simulink model "QAM_model1"  (Simulink 7.6)
settings: Solver=FixedStepDiscrete  SolverMode=SingleTasking  StartTime=0.0  StopTime=1  FixedStep=Ts  RelTol=1e-3  AbsTol=1e-6
PreLoadFcn:
  | fs=100000; Ts=1/fs; R=1000; T=1/R; fc=10000; M=16; A=20*sqrt(T/2);
undefined symbols (not defined in the file): get
libraries: commsink2 x2, commfilt2 x2, simulink x2, commrandsrc2 x1
settings Model: Creator=Lab220  LastModifiedBy=Sílvio
settings DataIOCC: LimitDataPoints=off  SignalLoggingName=sigsOut
settings OptimizationCC: BooleanDataType=off
settings DebuggingCC: SaveWithParameterizedLinksMsg=none  SignalResolutionControl=TryResolveAllWithWarning  SolverPrmCheckMsg=none  MultiTaskDSMMsg=warning  MultiTaskCondExecSysMsg=none  StrictBusMsg=None
settings HardwareCC: TargetUnknown=on
settings RTWCC: TemplateMakefile=grt_unix.tmf  IncludeERTFirstTime=on
settings GRTTargetCC: ModelReferenceCompliant=off  MatFileLogging=off

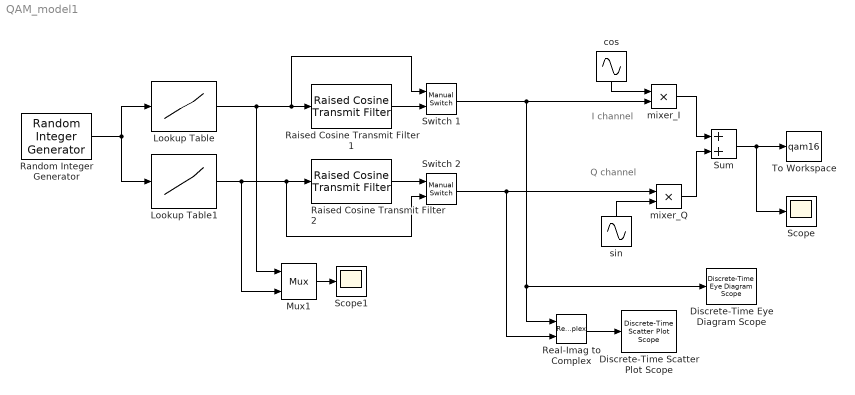
== system QAM_model1 ==
  note: I channel
  note: Q channel
  Discrete-Time Eye Diagram Scope : commsink2/Discrete-Time Eye Diagram Scope  Tag=EyeDiagram  SystemSampleTime=-1  sampPerSymb=100  offsetEye=0  symbPerTrace=2  numTraces=100  numNewFrames=4  LineStyles=-  LineColors=b  dupPoints=on  fading=on  render=on  AxisGrid=on  yMin=-4  yMax=4  inphaseLabel=In-phase Amplitude  quadratureLabel=Quadrature Amplitude  openScopeAtSimStart=on  dispDiagram=In-phase Only  FrameNumber=off  FigPos=get(0,'defaultfigureposition');  figTitle=Eye Diagram  block_type_=eye  numLinesMax=8
  Discrete-Time Scatter Plot Scope : commsink2/Discrete-Time Scatter Plot Scope  Tag=ScatterPlot  SystemSampleTime=-1  sampPerSymb=fs/R  offsetEye=0  numTraces=100  numNewFrames=100  LineMarkers=.  LineColors=b  fading=on  render=on  AxisGrid=on  xMin=-4  xMax=4  yMin=-4  yMax=4  inphaseLabel=In-phase Amplitude  quadratureLabel=Quadrature Amplitude  openScopeAtSimStart=on  FrameNumber=off  FigPos=get(0,'defaultfigureposition');  figTitle=Scatter Plot  numLinesMax=8  block_type_=scatter
  Lookup Table : Lookup_n-D  NumberOfTableDimensions=1  BreakpointsForDimension1=[0:15]  Table=[-3 -3 -3 -3 -1 -1 -1 -1 3 3 3 3 1 1 1 1]  InputSameDT=on
  Lookup Table1 : Lookup_n-D  NumberOfTableDimensions=1  BreakpointsForDimension1=[0:15]  Table=[-3 -1 3 1 -3 -1 3 1 -3 -1 3 1 -3 -1 3 1]  InputSameDT=on
  Mux1 : Mux  Inputs=2
  Raised Cosine Transmit Filter 1 : commfilt2/Raised Cosine Transmit Filter  DialogController=dspDDGCreate  DialogControllerArgs=DataTag1  SystemSampleTime=-1  filtType=Normal  D=4  R=0.5  sampMode=Mute  saveAsFlag=0  N=100  framing=Maintain input frame size  checkGain=Normalized  filterGain=1  checkCoeff=off  variableName=rcTxFilt  launchFVT=off  roundingMode=Floor  overflowMode=off
  Raised Cosine Transmit Filter 2 : commfilt2/Raised Cosine Transmit Filter  DialogController=dspDDGCreate  DialogControllerArgs=DataTag3  SystemSampleTime=-1  filtType=Normal  D=4  R=0.5  sampMode=Mute  saveAsFlag=0  N=100  framing=Maintain input frame size  checkGain=Normalized  filterGain=1  checkCoeff=off  variableName=rcTxFilt1  launchFVT=off  roundingMode=Floor  overflowMode=off
  Random Integer Generator : commrandsrc2/Random Integer Generator  SystemSampleTime=-1  mul=M  seed=randseed  Ts=T  frameBased=off  sampPerFrame=1  orient=off  outDataType=double
  Real-Imag to Complex : RealImagToComplex
  Scope : Scope
      settings: TickLabels=on  TimeRange=0.01  DataFormat=Array
  Scope1 : Scope
      settings: TickLabels=on  YMin=-4  YMax=4  DataFormat=Array
  Sum : Sum  SampleTime=Ts  SaturateOnIntegerOverflow=on  InputSameDT=on  OutDataTypeStr=Inherit: Same as first input
  Switch 1 : simulink/Signal Routing/Manual Switch  SystemSampleTime=-1  sw=0  action=0  varsize=off
  Switch 2 : simulink/Signal Routing/Manual Switch  SystemSampleTime=-1  sw=1  action=0  varsize=off
  To Workspace : ToWorkspace  VariableName=qam16  SampleTime=Ts  SaveFormat=Array
  cos : Sin  Frequency=2*pi*fc  Phase=pi/2  SampleTime=0
  mixer_I : Product  SampleTime=Ts  SaturateOnIntegerOverflow=on  InputSameDT=on  OutDataTypeStr=Inherit: Same as first input
  mixer_Q : Product  SampleTime=Ts  SaturateOnIntegerOverflow=on  InputSameDT=on  OutDataTypeStr=Inherit: Same as first input
  sin : Sin  Frequency=2*pi*fc  SampleTime=0
  wires:
  Raised Cosine Transmit Filter 2/1 -> Switch 2/1
  Raised Cosine Transmit Filter 1/1 -> Switch 1/2
  Mux1/1 -> Scope1/1
  Random Integer Generator/1 -> Lookup Table/1, Lookup Table1/1
  mixer_I/1 -> Sum/1
  mixer_Q/1 -> Sum/2
  sin/1 -> mixer_Q/2
  cos/1 -> mixer_I/1
  Sum/1 -> Scope/1, To Workspace/1
  Real-Imag to Complex/1 -> Discrete-Time Scatter Plot Scope/1
  Lookup Table/1 -> Mux1/1, Switch 1/1, Raised Cosine Transmit Filter 1/1
  Lookup Table1/1 -> Mux1/2, Raised Cosine Transmit Filter 2/1, Switch 2/2
  Switch 1/1 -> mixer_I/2, Discrete-Time Eye Diagram Scope/1, Real-Imag to Complex/1
  Switch 2/1 -> mixer_Q/1, Real-Imag to Complex/2
